simulink model "sim"  (R2015a)
settings: Solver=ode45  StartTime=0.0  StopTime=10.0  RelTol=1e-3
values from neighbouring files (symbols this model uses):
  CDMv = 0    [first.m]
  K1 = 10    [first.m]
  PLv = 1    [first.m]
  PRv = -0.9    [first.m]
  tau1 = 0.1    [first.m]
  th1_0 = 0    [first.m]
  th2_0 = -pi/4    (= -0.785398163397)    [first.m]
  th3_0 = -pi/4    (= -0.785398163397)    [first.m]
  th4_0 = pi/4    (= 0.785398163397)    [first.m]
  th5_0 = pi/4    (= 0.785398163397)    [first.m]
settings Model: Creator=max.sonzogni  LastModifiedBy=Max
settings DataIOCC: SaveFormat=Dataset
settings HardwareCC: ProdBitPerPointer=64  ProdLargestAtomicFloat=Float  ProdIntDivRoundTo=Zero  ProdEndianess=LittleEndian  ProdHWDeviceType=Specified
settings ModelReferenceCC: ModelReferenceMinAlgLoopOccurrences=on
settings GRTTargetCC: GeneratePreprocessorConditionals=Use local settings

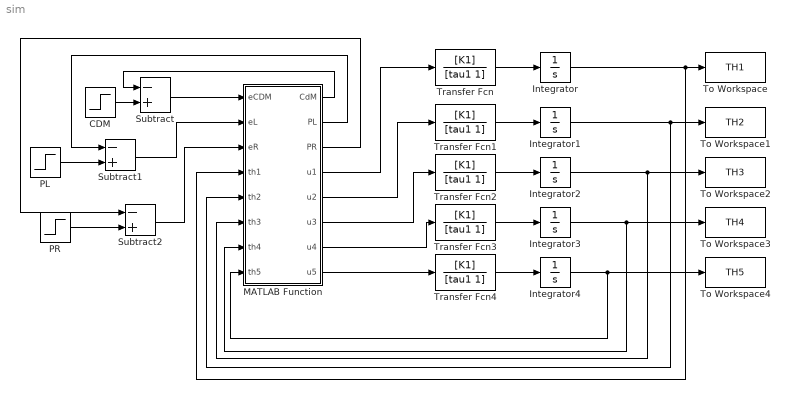
== system sim ==
  CDM : Step  Before=CDMv  After=CDMv  SampleTime=0
  Integrator : Integrator  InitialCondition=th1_0
  Integrator1 : Integrator  InitialCondition=th2_0
  Integrator2 : Integrator  InitialCondition=th3_0
  Integrator3 : Integrator  InitialCondition=th4_0
  Integrator4 : Integrator  InitialCondition=th5_0
  MATLAB Function : MATLAB Function  TreatAsAtomicUnit=on
      settings: PermitHierarchicalResolution=ParametersOnly
  PL : Step  Before=PLv  After=PLv  SampleTime=0
  PR : Step  Before=PRv  After=PRv  SampleTime=0
  Subtract : Sum  Inputs=-+
  Subtract1 : Sum  Inputs=-+
  Subtract2 : Sum  Inputs=-+
  To Workspace : ToWorkspace  VariableName=TH1  SampleTime=-1
  To Workspace1 : ToWorkspace  VariableName=TH2  SampleTime=-1
  To Workspace2 : ToWorkspace  VariableName=TH3  SampleTime=-1
  To Workspace3 : ToWorkspace  VariableName=TH4  SampleTime=-1
  To Workspace4 : ToWorkspace  VariableName=TH5  SampleTime=-1
  Transfer Fcn{,1..4} (5 alike) : TransferFcn  Numerator=[K1]  Denominator=[tau1 1]
  wires:
  CDM/1 -> Subtract/2
  Transfer Fcn/1 -> Integrator/1
  Integrator/1 -> To Workspace/1, MATLAB Function/4(th1)
  MATLAB Function/4(u1) -> Transfer Fcn/1
  Subtract/1 -> MATLAB Function/1(eCDM)
  PL/1 -> Subtract1/2
  Subtract1/1 -> MATLAB Function/2(eL)
  PR/1 -> Subtract2/2
  Subtract2/1 -> MATLAB Function/3(eR)
  MATLAB Function/1(CdM) -> Subtract/1
  MATLAB Function/2(PL) -> Subtract1/1
  MATLAB Function/3(PR) -> Subtract2/1
  MATLAB Function/5(u2) -> Transfer Fcn1/1
  Transfer Fcn1/1 -> Integrator1/1
  Integrator1/1 -> To Workspace1/1, MATLAB Function/5(th2)
  MATLAB Function/6(u3) -> Transfer Fcn2/1
  Transfer Fcn2/1 -> Integrator2/1
  Integrator2/1 -> MATLAB Function/6(th3), To Workspace2/1
  MATLAB Function/7(u4) -> Transfer Fcn3/1
  Transfer Fcn3/1 -> Integrator3/1
  Integrator3/1 -> To Workspace3/1, MATLAB Function/7(th4)
  MATLAB Function/8(u5) -> Transfer Fcn4/1
  Transfer Fcn4/1 -> Integrator4/1
  Integrator4/1 -> MATLAB Function/8(th5), To Workspace4/1

== matlab function sim/MATLAB Function ==
  data: CdM output; PL output; PR output; eCDM input; u1 output; eL input; eR input; th1 input; th2 input; th3 input; th4 input; th5 input; u2 output; u3 output; u4 output; u5 output
function [CdM,PL,PR,u1,u2,u3,u4,u5] = fcn(eCDM, eL, eR, th1, th2, th3, th4, th5)

le = 0.3; l1 = 0.7; l2 = 0.4; l3 = 0.3; l4 = 0.4; l5 = 0.3;
c1 = 0.6; c2 = 0.2; c3 = 0.15; c4 = 0.2; c5 = 0.15;
m1 = 20; m2 = 6; m3 = 4; m4 = 6; m5 = 4;

JL = [-l1*cos(th1)-(le/2)*sin(th1)+l2*sin(-th1+th2)+l3*sin(-th1+th2-th3) -l2*sin(-th1+th2)-l3*sin(-th1+th2-th3) l3*sin(-th1+th2-th3) 0 0];
JR = [-l1*cos(th1)+(le/2)*sin(th1)-l4*sin(-th1+th4)-l5*sin(-th1+th4-th5) 0 0 l4*sin(-th1+th4)+l5*sin(-th1+th4-th5) -l5*sin(-th1+th4-th5)];

cdm1 = [-c1*cos(th1) 0 0 0 0];
cdm2 = [-l1*cos(th1)-(le/2)*sin(th1)+c2*sin(-th1+th2) -c2*sin(-th1+th2) 0 0 0];
cdm3 = [-l1*cos(th1)-(le/2)*sin(th1)+l2*sin(-th1+th2)+c3*sin(-th1+th2-th3) -l2*sin(-th1+th2)-c3*sin(-th1+th2-th3) c3*sin(-th1+th2-th3) 0 0];
cdm4 = [-l1*cos(th1)+(le/2)*sin(th1)-c4*sin(-th1+th4) 0 0 c4*sin(-th1+th4) 0];
cdm5 = [-l1*cos(th1)+(le/2)*sin(th1)-l4*sin(-th1+th4)-c5*sin(-th1+th4-th5) 0 0 l4*sin(-th1+th4)+c5*sin(-th1+th4-th5) -c5*sin(-th1+th4-th5)];
Jcdm = (m1*cdm1+m2*cdm2+m3*cdm3+m4*cdm4+m5*cdm5)/(m1+m2+m3+m4+m5);

J1 = JR; J2 = JL; J3 = Jcdm;
e1 = eR; e2 = eL; e3 = eCDM;

P1 = eye(5) - pinv(J1)*J1;
P2 = eye(5) - pinv(J2)*J2;

th_1 = pinv(J1)*e1;
th_2 = pinv(J2*P1)*(e2-J2*th_1);
th_3 = pinv(J3*P2)*(e3-J3*th_2);

thetaP = th_1+th_2+th_3;
u1 = thetaP(1); u2 = thetaP(2); u3 = thetaP(3); u4 = thetaP(4); u5 = thetaP(5);

PL = -l1*sin(th1)+(le/2)*cos(th1)+l2*cos(-th1+th2)+l3*cos(-th1+th2-th3);
PR = -l1*sin(th1)-(le/2)*cos(th1)-l4*cos(-th1+th4)-l5*cos(-th1+th4-th5);

oc1 = -c1*sin(th1);
oc2 = -l1*sin(th1)+(le/2)*cos(th1)+c2*cos(-th1+th2);
ocL = -l1*sin(th1)+(le/2)*cos(th1)+l2*cos(-th1+th2)+c3*cos(-th1+th2-th3);
oc4 = -l1*sin(th1)-(le/2)*cos(th1)-c4*cos(-th1+th4);
ocR = -l1*sin(th1)-(le/2)*cos(th1)-l4*cos(-th1+th4)-c5*cos(-th1+th4-th5);
CdM = (m1*oc1+m2*oc2+m3*ocL+m4*oc4+m5*ocR)/(m1+m2+m3+m4+m5);

end
